simulink model "model_EV_pt1"  (R2022a)
settings: Solver=ode15s  StartTime=0.0  StopTime=tstop  MaxStep=0.001  RelTol=1e-3  EnableMultiTasking=on
undefined symbols (not defined in the file): D, F0, F1, F2, J, Km, La, M, Q, Qo, r_wheel, Ra, Rbatt, slope, SOC_max, SOC_min, Voc, xdot_o
libraries: fl_lib x38, nesl_utility x21, simulink x2, sdl_lib x1
settings Model: Creator=MathWorks  LastModifiedBy=cdjaolek
settings SolverCC: ZeroCrossControl=DisableAll  AlgebraicLoopSolver=TrustRegion
settings DataIOCC: LimitDataPoints=on  SaveFormat=Array  ReturnWorkspaceOutputs=off
settings OptimizationCC: ExpressionDepthLimit=2147483647  InitFltsAndDblsToZero=on  LifeSpan=inf
settings DebuggingCC: AlgebraicLoopMsg=none  SaveWithParameterizedLinksMsg=none  UnderspecifiedInitializationDetection=Classic  MergeDetectMultiDrivingBlocksExec=none  SignalResolutionControl=TryResolveAllWithWarning  SolverPrmCheckMsg=warning  UnconnectedInputMsg=warning  UnconnectedOutputMsg=warning  UnconnectedLineMsg=warning  StateNameClashWarn=warning  SFUnexpectedBacktrackingDiag=warning  SFNoUnconditionalDefaultTransitionDiag=warning  SFExecutionAtInitializationDiag=none  SFMachineParentedDataDiag=warning  ArithmeticOperatorsInVariantConditions=warning
settings HardwareCC: ProdBitPerPointer=32  ProdBitPerSizeT=32  ProdBitPerPtrDiffT=32  ProdLargestAtomicFloat=None  ProdIntDivRoundTo=Undefined  ProdEndianess=Unspecified  ProdWordSize=32  ProdHWDeviceType=32-bit Generic
settings ModelReferenceCC: PropagateSignalLabelsOutOfModel=off
settings SFSimCC: SimUseLocalCustomCode=off  CustomCodeUndefinedFunction=UseInterfaceOnly
settings RTWCC: RTWUseLocalCustomCode=off
settings CodeAppCC: StateflowObjectComments=on
settings GRTTargetCC: TargetFcnLib=ansi_tfl_tmw.mat  TargetLangStandard=C89/C90 (ANSI)  CombineOutputUpdateFcns=off  GRTInterface=on
settings ConfigComp: CovMetricSettings=dw  CovSaveCumulativeToWorkspaceVar=on  CovSaveSingleToWorkspaceVar=on  CovExternalEMLEnable=off
settings SimscapeCC: SimscapeNormalizeSystem=off

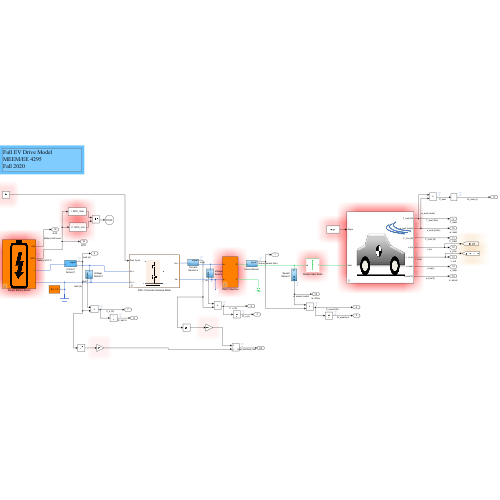
[thumbnail: Simulink's stored preview of the top-level diagram]
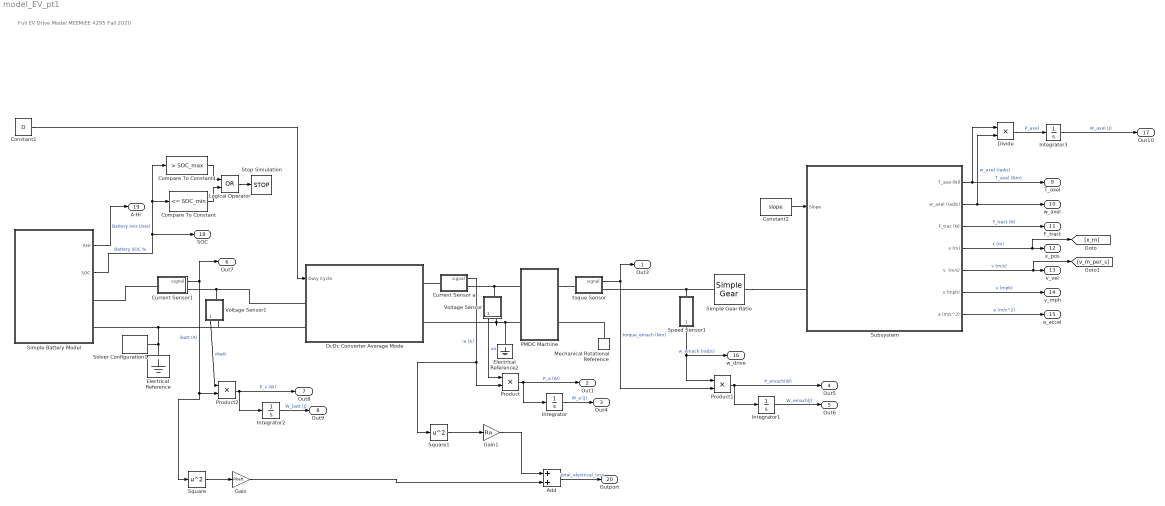
== system model_EV_pt1 ==
  note: Full EV Drive Model
      | MEEM/EE 4295
      | Fall 2020
  Add : Sum
  Compare To Constant : simulink/Logic and Bit Operations/Compare To Constant  relop=<=  const=SOC_min  OutDataTypeStr=boolean
  Compare To Constant1 : simulink/Logic and Bit Operations/Compare To Constant  relop=>  const=SOC_max  OutDataTypeStr=boolean
  Constant1 : Constant  Value=D
  Constant2 : Constant  Value=slope
  Current Sensor a : Subsystem
  Current Sensor1 : Subsystem
  DcDc Converter Average Mode : Subsystem
      mask help: Two Quadrant Dc-Dc convereter - average mode (no switching)
      mask Display: image('$imagefile'); % Use "Edit Image" on toolstrip to change.
  Divide : Product
  Electrical Reference : fl_lib/Electrical/Electrical Elements/Electrical Reference
      settings: SourceProductBaseCode=PW,SS,VE
  Electrical Reference2 : fl_lib/Electrical/Electrical Elements/Electrical Reference
      settings: SourceProductBaseCode=PW,SS,VE
  Gain : Gain  Gain=Rbatt
  Gain1 : Gain  Gain=Ra
  Integrator{,1..3} (4 alike) : Integrator
  Logical Operator : Logic  Operator=OR  AllPortsSameDT=off  OutDataTypeStr=boolean
  Mechanical Rotational Reference : fl_lib/Mechanical/Rotational Elements/Mechanical Rotational Reference
      settings: SourceProductBaseCode=PW,SS,VE
  PMDC Machine : Subsystem  mask{Km=Km, Ra=Ra, La=La, J=J, B=1e-6}
      mask prompts: Km "Motor Constant (Nm/A)"; Ra "Armature Resistance (Ohm)"; La "Armature Inductance (H)"; J "Motor Inertia (kg m^2)"; B "Motor Damping (N*m/(rad/s))"
      mask help: Permanent Magnet DC Motor
  Product : Product
  Product1 : Product
  Product2 : Product
  Simple Battery Model : Subsystem  mask{Voc=Voc, Rbatt=Rbatt, Q=Q, Qo=Qo}
      mask prompts: Voc "Open Circuit Voltage"; Rbatt "Battery  Resistance"; Q "AHr Capacity"; Qo "Initial AHr Used"
      mask help: Simple Battery Model
      mask Display: image('$imagefile'); % Use "Edit Image" on toolstrip to change.
  Simple Gear Ratio : sdl_lib/Gears/Simple Gear  ratio=GR  rotation_direction=3-2*(1)  friction_model=sdl.enum.gear_efficiencies_load.off  T_noload=0.1 N*m  T_nom=5 N*m  efficiency_nom=0.8  efficiency=0.8  temperature_TLU=[280, 300, 320] K  load_TLU=[1, 5, 10] N*m  efficiency_TLU=[.95, .9, .85]  efficiency_TLU2=[.85, .8, .75; .95, .9, .85; .85, .8, .7]  w_thr=0.01 rad/s  pwr_thr=0.001 W  backlash_model=sdl.enum.backlashModel.Off  backlash_distance=1e-3 mm  x0=0 mm  r_base=0.1 m  hardstop_model=simscape.enum.hardstop.smooth  transition=1e-4 mm  backlash_stiffness=1e7 N/m  backlash_damping=1e6 N*s/m  e=0  v_tol=0.001 m/s  mu_visc=[0, 0] N*m/(rad/s)  enable_faults=simscape.enum.onoff.off  efficiency_fault=0.05  external_fault=simscape.enum.onoff.off  temporal_fault=simscape.enum.onoff.off  fault_time=5 s  fault_angles=pi / 12 rad  report_fault=(1)-1  thermal_mass=50 J/K  temperature_specify=off  temperature_priority=High  temperature=300 K  temperature_nominal_specify=off  temperature_nominal_unit=K  temperature_nominal_value=1  x_backlash_specify=off  x_backlash_priority=None  x_backlash=0 mm  x_backlash_nominal_specify=off  x_backlash_nominal_unit=mm  x_backlash_nominal_value=1  f_hardstop_specify=off  f_hardstop_priority=None  f_hardstop=0 N  f_hardstop_nominal_specify=off  f_hardstop_nominal_unit=N  f_hardstop_nominal_value=1  v_backlash_specify=off  v_backlash_priority=None  v_backlash=0 m/s  v_backlash_nominal_specify=off  v_backlash_nominal_unit=m/s  v_backlash_nominal_value=1
  Solver Configuration1 : nesl_utility/Solver Configuration  PhysicalDomain=network_engine_domain  SubClassName=solver  LeftPortType=input  RightPortType=generic  Tones=[]  Harmonics=[]  SimulateNoise=off  Profile=off  UseLocalSampling=off  EnableSwitchedLinearOptims=on  FrequencyDomain=off  UseCCode=off  RelTol=0.001  AbsTol=1e-06  MinStep=1e-09  ToWorkspace=off  RevertToSquareIcSolve=off  NumHomotopyIterations=100  PhasorMode=off  PhasorModeNumHarmonics=1  IndexReductionMethod=DerivativeReplacement  DoDC=off  ResidualTolerance=1e-9  UseLocalSolver=off  LocalSolverChoice=NE_TRAPEZOIDAL_ADVANCER  LocalSolverSampleTime=1e-7  DoFixedCost=off  MaxNonlinIter=3  MaxModeIter=2  ComputeImpulses=off  ImpulseIterations=2  LinearAlgebra=Sparse  LinearAlgebraNumThread=0  EquationFormulation=NE_TIME_EF  DelaysMemoryBudget=1024  AutomaticFiltering=on  FilteringTimeConstant=0.001  PartitionStorageMethod=AS_NEEDED  PartitionMemoryBudget=1024  PartitionMethod=FAST
      settings: SourceProductBaseCode=SS,PW,VE
  Speed Sensor1 : Subsystem
  Square : Math  Operator=square
  Square1 : Math  Operator=square
  Stop Simulation : Stop
  Subsystem : Subsystem  mask{M=M, r_wheel=r_wheel, F0=F0, F1=F1, F2=F2, xdot_o=xdot_o}
      mask prompts: M "Vehicle Mass (kg)"; r_wheel "Wheel Radius (m)"; F0 "Rolling resistance coefficient, a [N]:"; F1 "Rolling and driveline resistance coefficient, b [N*s/m]:"; F2 "Aerodynamic drag coefficient, c [N*s^2/m^2]:"; xdot_o "Initial velocity, xdot_o [m/s]:"
      mask help: Simple vehicle dynamics model.
      mask Display: image('$imagefile'); % Use "Edit Image" on toolstrip to change.
  Voltage Sensor : Subsystem
  Voltage Sensor1 : Subsystem
  toque Sensor : Subsystem
  Out3 : Outport
  Out1 : Outport  Port=2
  Out4 : Outport  Port=3
  Out5 : Outport  Port=4
  Out6 : Outport  Port=5
  Out7 : Outport  Port=6
  Out8 : Outport  Port=7
  Out9 : Outport  Port=8
  T_axel : Outport  Port=9
  w_axel : Outport  Port=10
  F_tract : Outport  Port=11
  x_pos : Outport  Port=12
  v_vel : Outport  Port=13
  v_mph : Outport  Port=14
  a_accel : Outport  Port=15
  w_drive : Outport  Port=16
  Out10 : Outport  Port=17
  SOC : Outport  Port=18
  A-Hr : Outport  Port=19
  Outport : Outport  Port=20
  wires:
  Current Sensor a/1(signal) -> Square1/1, Product/2  "ia (A)"
  toque Sensor/1(signal) -> Out3/1, Product1/2  "torque_emach (Nm)"
  Voltage Sensor/1(signal) -> Product/1  "va"
  Product/1 -> Integrator/1, Out1/1  "P_a (W)"
  Integrator/1 -> Out4/1  "W_a (J)"
  Product1/1 -> Integrator1/1, Out5/1  "P_emach(W)"
  Integrator1/1 -> Out6/1  "W_emach(J)"
  Integrator2/1 -> Out9/1  "W_batt (J)"
  Product2/1 -> Integrator2/1, Out8/1  "P_s (W)"
  Voltage Sensor1/1(signal) -> Product2/1  "vbatt"
  Current Sensor1/1(signal) -> Out7/1, Square/1, Product2/2  "ibatt (A)"
  Constant1/1 -> DcDc Converter Average Mode/1(Duty Cycle)
  Speed Sensor1/1(rad/s) -> Product1/1, w_drive/1  "w_emach (rad/s)"
  Subsystem/2(w_axel (rad/s)) -> w_axel/1, Divide/2  "w_axel (rad/s)"
  Constant2/1 -> Subsystem/1(Slope)
  Subsystem/5(v  (m/s)) -> [v_m_per_s], v_vel/1  "v (m/s)"
  Subsystem/6(v (mph)) -> v_mph/1  "v (mph)"
  Subsystem/1(T_axe (N)l) -> T_axel/1, Divide/1  "T_axel (Nm)"
  Subsystem/3(F_trac (N)) -> F_tract/1  "F_tract (N)"
  Divide/1 -> Integrator3/1  "P_axel"
  Integrator3/1 -> Out10/1  "W_axel (J)"
  Subsystem/7(a (m/s^2)) -> a_accel/1  "a (m/s^2)"
  Subsystem/4(x (m)) -> [x_m], x_pos/1  "x (m)"
  Simple Battery Model/1(AHr) -> A-Hr/1  "Battery AHr Used"
  Logical Operator/1 -> Stop Simulation/1
  Compare To Constant1/1 -> Logical Operator/1
  Simple Battery Model/2(SOC) -> Compare To Constant/1, Compare To Constant1/1, SOC/1  "Battery SOC %"
  Compare To Constant/1 -> Logical Operator/2
  Add/1 -> Outport/1  "total_electrical_loss"
  Square/1 -> Gain/1
  Square1/1 -> Gain1/1
  Gain/1 -> Add/2
  Gain1/1 -> Add/1
  connections:
  Mechanical Rotational Reference/LConn1 -- PMDC Machine/RConn2
  Voltage Sensor/LConn1 -- PMDC Machine/LConn1 -- Current Sensor a/RConn1
  PMDC Machine/RConn1 -- toque Sensor/LConn1
  Solver Configuration1/RConn1 -- Electrical Reference/LConn1 -- Voltage Sensor1/RConn1 -- DcDc Converter Average Mode/LConn2 -- Simple Battery Model/RConn2
  Current Sensor a/LConn1 -- DcDc Converter Average Mode/RConn1
  Current Sensor1/LConn1 -- Simple Battery Model/RConn1
  DcDc Converter Average Mode/LConn1 -- Voltage Sensor1/LConn1 -- Current Sensor1/RConn1
  PMDC Machine/LConn2 -- Electrical Reference2/LConn1 -- Voltage Sensor/RConn1 -- DcDc Converter Average Mode/RConn2
  Speed Sensor1/LConn1 -- Simple Gear Ratio/LConn1 -- toque Sensor/RConn1
  Simple Gear Ratio/RConn1 -- Subsystem/LConn1

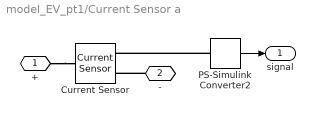
== system model_EV_pt1/Current Sensor a ==
  Current Sensor : fl_lib/Electrical/Electrical Sensors/Current Sensor
      settings: SourceProductBaseCode=PW,SS,VE
  PS-Simulink Converter2 : nesl_utility/PS-Simulink Converter  PhysicalDomain=network_engine_domain  SubClassName=ps_output  LeftPortType=input  RightPortType=output  PseudoPeriodic=off  Frequencies=[]  VectorFormat=1-D array  Unit=1  AffineConversion=off
      settings: SourceProductBaseCode=SS,PW,VE
  + : PMIOPort  Side=Left
  - : PMIOPort  Port=2  Side=Right
  signal : Outport
  wires:
  PS-Simulink Converter2/1 -> signal/1
  connections:
  PS-Simulink Converter2/LConn1 -- Current Sensor/RConn1
  +/RConn1 -- Current Sensor/LConn1
  -/RConn1 -- Current Sensor/RConn2

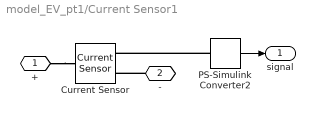
== system model_EV_pt1/Current Sensor1 ==
  Current Sensor : fl_lib/Electrical/Electrical Sensors/Current Sensor
      settings: SourceProductBaseCode=PW,SS,VE
  PS-Simulink Converter2 : nesl_utility/PS-Simulink Converter  PhysicalDomain=network_engine_domain  SubClassName=ps_output  LeftPortType=input  RightPortType=output  PseudoPeriodic=off  Frequencies=[]  VectorFormat=1-D array  Unit=1  AffineConversion=off
      settings: SourceProductBaseCode=SS,PW,VE
  + : PMIOPort  Side=Left
  - : PMIOPort  Port=2  Side=Right
  signal : Outport
  wires:
  PS-Simulink Converter2/1 -> signal/1
  connections:
  PS-Simulink Converter2/LConn1 -- Current Sensor/RConn1
  +/RConn1 -- Current Sensor/LConn1
  -/RConn1 -- Current Sensor/RConn2

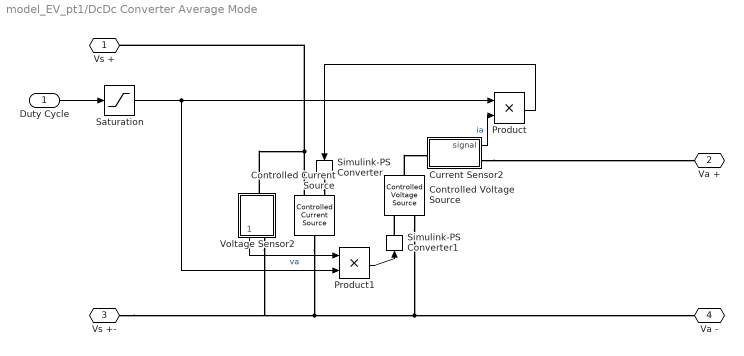
== system model_EV_pt1/DcDc Converter Average Mode ==
  Duty Cycle : Inport
  Controlled Current Source : fl_lib/Electrical/Electrical Sources/Controlled Current Source
      settings: SourceProductBaseCode=PW,SS,VE
  Controlled Voltage Source : fl_lib/Electrical/Electrical Sources/Controlled Voltage Source
      settings: SourceProductBaseCode=PW,SS,VE
  Current Sensor2 : Subsystem
  Product : Product
  Product1 : Product
  Saturation : Saturate  UpperLimit=1  LowerLimit=0
  Simulink-PS Converter : nesl_utility/Simulink-PS Converter  PhysicalDomain=network_engine_domain  SubClassName=ps_input  LeftPortType=input  RightPortType=output  PseudoPeriodic=off  Frequencies=[]  NoiseDistribution=none  NoiseParameters=[]  Unit=1  AffineConversion=off  FilteringAndDerivatives=provide  SimscapeFilterOrder=1  InputFilterTimeConstant=0.001  UdotUserProvided=0
      settings: SourceProductBaseCode=SS,PW,VE
  Simulink-PS Converter1 : nesl_utility/Simulink-PS Converter  PhysicalDomain=network_engine_domain  SubClassName=ps_input  LeftPortType=input  RightPortType=output  PseudoPeriodic=off  Frequencies=[]  NoiseDistribution=none  NoiseParameters=[]  Unit=1  AffineConversion=off  FilteringAndDerivatives=provide  SimscapeFilterOrder=1  InputFilterTimeConstant=0.001  UdotUserProvided=0
      settings: SourceProductBaseCode=SS,PW,VE
  Voltage Sensor2 : Subsystem
  Vs + : PMIOPort  Side=Left
  Va + : PMIOPort  Port=2  Side=Right
  Vs +- : PMIOPort  Port=3  Side=Left
  Va - : PMIOPort  Port=4  Side=Right
  wires:
  Product1/1 -> Simulink-PS Converter1/1
  Duty Cycle/1 -> Saturation/1
  Voltage Sensor2/1(signal) -> Product1/1  "va"
  Product/1 -> Simulink-PS Converter/1
  Current Sensor2/1(signal) -> Product/2  "ia"
  Saturation/1 -> Product1/2, Product/1
  connections:
  Controlled Current Source/RConn2 -- Vs +/RConn1 -- Voltage Sensor2/LConn1
  Simulink-PS Converter/RConn1 -- Controlled Current Source/RConn1
  Simulink-PS Converter1/RConn1 -- Controlled Voltage Source/RConn1
  Controlled Voltage Source/LConn1 -- Current Sensor2/LConn1
  Current Sensor2/RConn1 -- Va +/RConn1
  Controlled Voltage Source/RConn2 -- Voltage Sensor2/RConn1 -- Vs +-/RConn1 -- Controlled Current Source/LConn1 -- Va -/RConn1

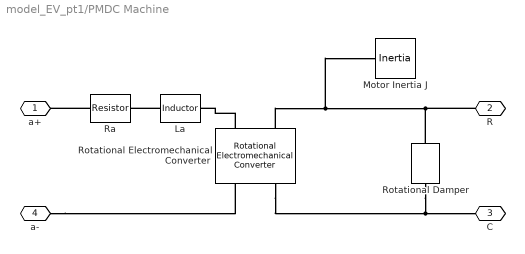
== system model_EV_pt1/PMDC Machine ==
  La : fl_lib/Electrical/Electrical Elements/Inductor  l=La H  r=0 Ohm  g=1e-09 1/Ohm  i_specify=off  i_priority=None  i=0 A  i_nominal_specify=off  i_nominal_unit=A  i_nominal_value=1  v_specify=off  v_priority=None  v=0 V  v_nominal_specify=off  v_nominal_unit=V  v_nominal_value=1  i_L_specify=on  i_L_priority=High  i_L=0 A  i_L_nominal_specify=off  i_L_nominal_unit=A  i_L_nominal_value=1
      settings: SourceProductBaseCode=PW,SS,VE
  Motor Inertia J : fl_lib/Mechanical/Rotational Elements/Inertia  inertia=J kg*m^2  num_ports=foundation.enum.numPorts2.one  w_specify=on  w_priority=High  w=0 rad/s  w_nominal_specify=off  w_nominal_unit=rad/s  w_nominal_value=1  t_specify=off  t_priority=None  t=0 N*m  t_nominal_specify=off  t_nominal_unit=N*m  t_nominal_value=1
      settings: SourceProductBaseCode=PW,SS,VE
  Ra : fl_lib/Electrical/Electrical Elements/Resistor  Tag=Factory Generic  R=Ra Ohm  i_specify=off  i_priority=None  i=0 A  i_nominal_specify=off  i_nominal_unit=A  i_nominal_value=1  v_specify=off  v_priority=None  v=0 V  v_nominal_specify=off  v_nominal_unit=V  v_nominal_value=1
      settings: SourceProductBaseCode=PW,SS,VE
  Rotational Damper : fl_lib/Mechanical/Rotational Elements/Rotational Damper  D=B N*m/(rad/s)  w_specify=off  w_priority=None  w=0 rad/s  w_nominal_specify=off  w_nominal_unit=rad/s  w_nominal_value=1  t_specify=off  t_priority=None  t=0 N*m  t_nominal_specify=off  t_nominal_unit=N*m  t_nominal_value=1
      settings: SourceProductBaseCode=PW,SS,VE
  Rotational Electromechanical Converter : fl_lib/Electrical/Electrical Elements/Rotational Electromechanical Converter  K=Km V/(rad/s)  i_specify=off  i_priority=None  i=0 A  i_nominal_specify=off  i_nominal_unit=A  i_nominal_value=1  v_specify=off  v_priority=None  v=0 V  v_nominal_specify=off  v_nominal_unit=V  v_nominal_value=1  t_specify=off  t_priority=None  t=0 N*m  t_nominal_specify=off  t_nominal_unit=N*m  t_nominal_value=1  w_specify=off  w_priority=None  w=0 rad/s  w_nominal_specify=off  w_nominal_unit=rad/s  w_nominal_value=1
      settings: SourceProductBaseCode=PW,SS,VE
  a+ : PMIOPort  Side=Left
  R : PMIOPort  Port=2  Side=Right
  C : PMIOPort  Port=3  Side=Right
  a- : PMIOPort  Port=4  Side=Left
  connections:
  Rotational Electromechanical Converter/LConn1 -- La/RConn1
  a-/RConn1 -- Rotational Electromechanical Converter/RConn1
  Ra/LConn1 -- a+/RConn1
  La/LConn1 -- Ra/RConn1
  Rotational Electromechanical Converter/LConn2 -- Motor Inertia J/LConn1 -- R/RConn1 -- Rotational Damper/LConn1
  Rotational Electromechanical Converter/RConn2 -- C/RConn1 -- Rotational Damper/RConn1

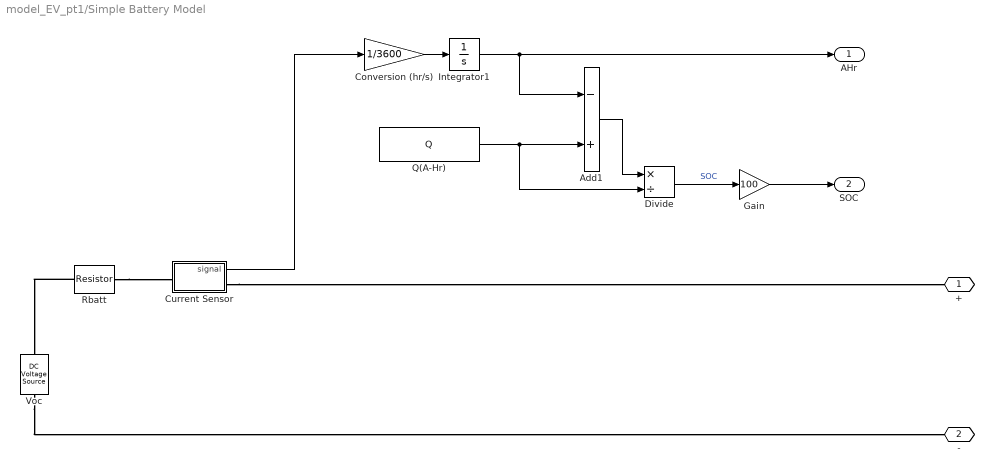
== system model_EV_pt1/Simple Battery Model ==
  Add1 : Sum  Inputs=-+
  Conversion (hr/s) : Gain  Gain=1/3600
  Current Sensor : Subsystem
  Divide : Product  Inputs=*/
  Gain : Gain  Gain=100
  Integrator1 : Integrator  InitialCondition=Qo  UpperSaturationLimit=Q*1.5  LowerSaturationLimit=0
  Q(A-Hr) : Constant  Value=Q
  Rbatt : fl_lib/Electrical/Electrical Elements/Resistor  R=Rbatt Ohm  i_specify=off  i_priority=None  i=0 A  i_nominal_specify=off  i_nominal_unit=A  i_nominal_value=1  v_specify=off  v_priority=None  v=0 V  v_nominal_specify=off  v_nominal_unit=V  v_nominal_value=1
      settings: SourceProductBaseCode=PW,SS,VE
  Voc : fl_lib/Electrical/Electrical Sources/DC Voltage Source  v0=Voc V
      settings: SourceProductBaseCode=PW,SS,VE
  + : PMIOPort  Side=Right
  - : PMIOPort  Port=2  Side=Right
  AHr : Outport
  SOC : Outport  Port=2
  wires:
  Integrator1/1 -> AHr/1, Add1/1
  Conversion (hr/s)/1 -> Integrator1/1
  Add1/1 -> Divide/1
  Divide/1 -> Gain/1  "SOC"
  Q(A-Hr)/1 -> Add1/2, Divide/2
  Gain/1 -> SOC/1
  Current Sensor/1(signal) -> Conversion (hr/s)/1
  connections:
  Rbatt/RConn1 -- Current Sensor/LConn1
  Current Sensor/RConn1 -- +/RConn1
  Rbatt/LConn1 -- Voc/LConn1
  Voc/RConn1 -- -/RConn1

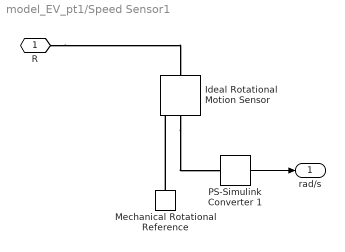
== system model_EV_pt1/Speed Sensor1 ==
  Ideal Rotational Motion Sensor : fl_lib/Mechanical/Mechanical Sensors/Ideal Rotational Motion Sensor  wrap_angle=simscape.enum.onoff.off  offset=0 rad
      settings: SourceProductBaseCode=PW,SS,VE
  Mechanical Rotational Reference : fl_lib/Mechanical/Rotational Elements/Mechanical Rotational Reference
      settings: SourceProductBaseCode=PW,SS,VE
  PS-Simulink Converter 1 : nesl_utility/PS-Simulink Converter  PhysicalDomain=network_engine_domain  SubClassName=ps_output  LeftPortType=input  RightPortType=output  PseudoPeriodic=off  Frequencies=[]  VectorFormat=1-D array  Unit=rad/s  AffineConversion=off
      settings: SourceProductBaseCode=SS,PW,VE
  R : PMIOPort  Side=Left
  rad/s : Outport
  wires:
  PS-Simulink Converter 1/1 -> rad/s/1
  connections:
  Ideal Rotational Motion Sensor/RConn2 -- PS-Simulink Converter 1/LConn1
  R/RConn1 -- Ideal Rotational Motion Sensor/LConn1
  Mechanical Rotational Reference/LConn1 -- Ideal Rotational Motion Sensor/RConn1

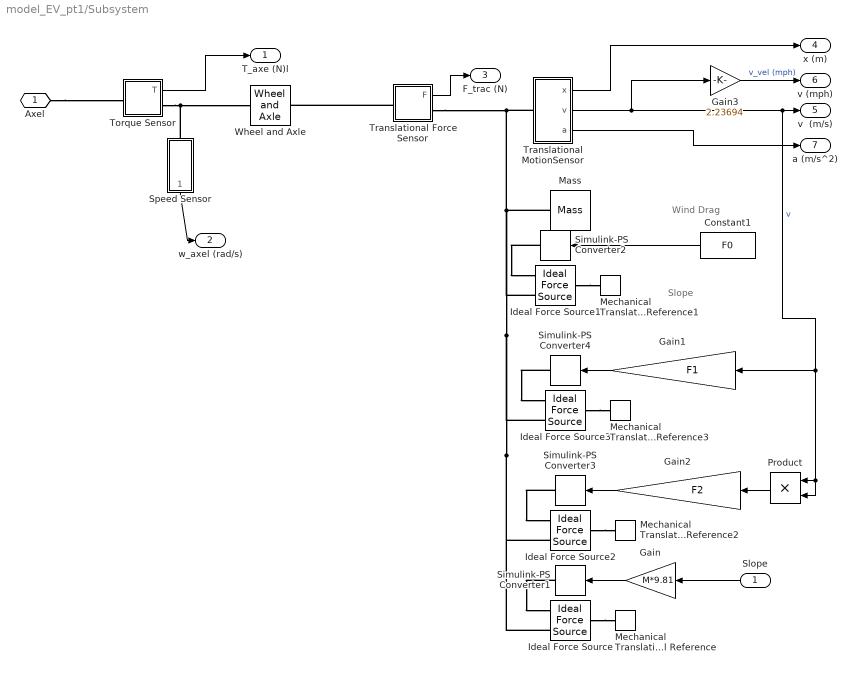
== system model_EV_pt1/Subsystem ==
  note: Wind Drag
  note: Slope
  Slope : Inport
  Constant1 : Constant  Value=F0
  Gain : Gain  Gain=M*9.81
  Gain1 : Gain  Gain=F1
  Gain2 : Gain  Gain=F2
  Gain3 : Gain  Gain=2.23694
  Ideal Force Source{,1..3} (4 alike) : fl_lib/Mechanical/Mechanical Sources/Ideal Force Source
      settings: SourceProductBaseCode=PW,SS,VE
  Mass : fl_lib/Mechanical/Translational Elements/Mass  mass=M kg  num_ports=foundation.enum.numPorts2.one  v_specify=on  v_priority=High  v=xdot_o m/s  v_nominal_specify=off  v_nominal_unit=m/s  v_nominal_value=1  f_specify=off  f_priority=None  f=0 N  f_nominal_specify=off  f_nominal_unit=N  f_nominal_value=1
      settings: SourceProductBaseCode=PW,SS,VE
  Mechanical Translational Reference{,1..3} (4 alike) : fl_lib/Mechanical/Translational Elements/Mechanical Translational Reference
      settings: SourceProductBaseCode=PW,SS,VE
  Product : Product  RndMeth=Zero
  Simulink-PS Converter{1..4} (4 alike) : nesl_utility/Simulink-PS Converter  PhysicalDomain=network_engine_domain  SubClassName=ps_input  LeftPortType=input  RightPortType=output  PseudoPeriodic=off  Frequencies=[]  NoiseDistribution=none  NoiseParameters=[]  Unit=1  AffineConversion=off  FilteringAndDerivatives=zero  SimscapeFilterOrder=1  InputFilterTimeConstant=.001  UdotUserProvided=[]
      settings: SourceProductBaseCode=SS,PW,VE
  Speed Sensor : Subsystem
  Torque Sensor : Subsystem
  Translational Force Sensor : Subsystem
  Translational MotionSensor : Subsystem
  Wheel and Axle : fl_lib/Mechanical/Mechanisms/Wheel and Axle  Tag=Factory Generic  R=r_wheel m  or=1  t_specify=off  t_priority=None  t=0 N*m  t_nominal_specify=off  t_nominal_unit=N*m  t_nominal_value=1  f_specify=off  f_priority=None  f=0 N  f_nominal_specify=off  f_nominal_unit=N  f_nominal_value=1
      settings: SourceProductBaseCode=PW,SS,VE
  Axel : PMIOPort  Side=Left
  T_axe (N)l : Outport
  w_axel (rad/s) : Outport  Port=2
  F_trac (N) : Outport  Port=3
  x (m) : Outport  Port=4
  v  (m/s) : Outport  Port=5
  v (mph) : Outport  Port=6
  a (m/s^2) : Outport  Port=7
  wires:
  Product/1 -> Gain2/1
  Translational MotionSensor/2(v) -> Gain1/1, Product/2, Product/1, v  (m/s)/1, Gain3/1  "v"
  Speed Sensor/1(rad/s) -> w_axel (rad/s)/1
  Gain/1 -> Simulink-PS Converter1/1
  Gain2/1 -> Simulink-PS Converter3/1
  Torque Sensor/1(T) -> T_axe (N)l/1
  Translational MotionSensor/1(x) -> x (m)/1
  Translational MotionSensor/3(a) -> a (m/s^2)/1
  Translational Force Sensor/1(F) -> F_trac (N)/1
  Slope/1 -> Gain/1
  Gain3/1 -> v (mph)/1  "v_vel (mph)"
  Constant1/1 -> Simulink-PS Converter2/1
  Gain1/1 -> Simulink-PS Converter4/1
  connections:
  Ideal Force Source1/LConn1 -- Mechanical Translational Reference1/LConn1
  Mass/LConn1 -- Ideal Force Source3/RConn2 -- Ideal Force Source/RConn2 -- Ideal Force Source2/RConn2 -- Ideal Force Source1/RConn2 -- Translational MotionSensor/LConn1 -- Translational Force Sensor/RConn1
  Ideal Force Source2/LConn1 -- Mechanical Translational Reference2/LConn1
  Torque Sensor/RConn1 -- Wheel and Axle/LConn1 -- Speed Sensor/LConn1
  Simulink-PS Converter1/RConn1 -- Ideal Force Source/RConn1
  Simulink-PS Converter2/RConn1 -- Ideal Force Source1/RConn1
  Ideal Force Source/LConn1 -- Mechanical Translational Reference/LConn1
  Translational Force Sensor/LConn1 -- Wheel and Axle/RConn1
  Simulink-PS Converter3/RConn1 -- Ideal Force Source2/RConn1
  Axel/RConn1 -- Torque Sensor/LConn1
  Simulink-PS Converter4/RConn1 -- Ideal Force Source3/RConn1
  Ideal Force Source3/LConn1 -- Mechanical Translational Reference3/LConn1

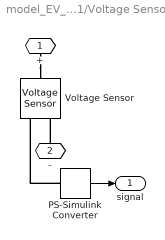
== system model_EV_pt1/Voltage Sensor ==
  PS-Simulink Converter : nesl_utility/PS-Simulink Converter  PhysicalDomain=network_engine_domain  SubClassName=ps_output  LeftPortType=input  RightPortType=output  PseudoPeriodic=off  Frequencies=[]  VectorFormat=1-D array  Unit=1  AffineConversion=off
      settings: SourceProductBaseCode=SS,PW,VE
  Voltage Sensor : fl_lib/Electrical/Electrical Sensors/Voltage Sensor
      settings: SourceProductBaseCode=PW,SS,VE
  + : PMIOPort  Side=Left
  - : PMIOPort  Port=2  Side=Right
  signal : Outport
  wires:
  PS-Simulink Converter/1 -> signal/1
  connections:
  PS-Simulink Converter/LConn1 -- Voltage Sensor/RConn1
  +/RConn1 -- Voltage Sensor/LConn1
  -/RConn1 -- Voltage Sensor/RConn2

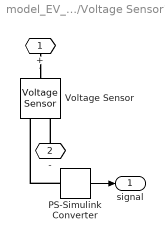
== system model_EV_pt1/Voltage Sensor1 ==
  PS-Simulink Converter : nesl_utility/PS-Simulink Converter  PhysicalDomain=network_engine_domain  SubClassName=ps_output  LeftPortType=input  RightPortType=output  PseudoPeriodic=off  Frequencies=[]  VectorFormat=1-D array  Unit=1  AffineConversion=off
      settings: SourceProductBaseCode=SS,PW,VE
  Voltage Sensor : fl_lib/Electrical/Electrical Sensors/Voltage Sensor
      settings: SourceProductBaseCode=PW,SS,VE
  + : PMIOPort  Side=Left
  - : PMIOPort  Port=2  Side=Right
  signal : Outport
  wires:
  PS-Simulink Converter/1 -> signal/1
  connections:
  PS-Simulink Converter/LConn1 -- Voltage Sensor/RConn1
  +/RConn1 -- Voltage Sensor/LConn1
  -/RConn1 -- Voltage Sensor/RConn2

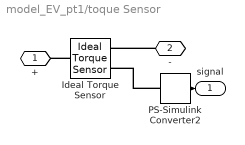
== system model_EV_pt1/toque Sensor ==
  Ideal Torque Sensor : fl_lib/Mechanical/Mechanical Sensors/Ideal Torque Sensor
      settings: SourceProductBaseCode=PW,SS,VE
  PS-Simulink Converter2 : nesl_utility/PS-Simulink Converter  PhysicalDomain=network_engine_domain  SubClassName=ps_output  LeftPortType=input  RightPortType=output  PseudoPeriodic=off  Frequencies=[]  VectorFormat=1-D array  Unit=1  AffineConversion=off
      settings: SourceProductBaseCode=SS,PW,VE
  + : PMIOPort  Side=Left
  - : PMIOPort  Port=2  Side=Right
  signal : Outport
  wires:
  PS-Simulink Converter2/1 -> signal/1
  connections:
  Ideal Torque Sensor/LConn1 -- +/RConn1
  -/RConn1 -- Ideal Torque Sensor/RConn1
  PS-Simulink Converter2/LConn1 -- Ideal Torque Sensor/RConn2

== system model_EV_pt1/DcDc Converter Average Mode/Current Sensor2 ==
  Current Sensor : fl_lib/Electrical/Electrical Sensors/Current Sensor
      settings: SourceProductBaseCode=PW,SS,VE
  PS-Simulink Converter2 : nesl_utility/PS-Simulink Converter  PhysicalDomain=network_engine_domain  SubClassName=ps_output  LeftPortType=input  RightPortType=output  PseudoPeriodic=off  Frequencies=[]  VectorFormat=1-D array  Unit=1  AffineConversion=off
      settings: SourceProductBaseCode=SS,PW,VE
  + : PMIOPort  Side=Left
  - : PMIOPort  Port=2  Side=Right
  signal : Outport
  wires:
  PS-Simulink Converter2/1 -> signal/1
  connections:
  PS-Simulink Converter2/LConn1 -- Current Sensor/RConn1
  +/RConn1 -- Current Sensor/LConn1
  -/RConn1 -- Current Sensor/RConn2

== system model_EV_pt1/DcDc Converter Average Mode/Voltage Sensor2 ==
  PS-Simulink Converter : nesl_utility/PS-Simulink Converter  PhysicalDomain=network_engine_domain  SubClassName=ps_output  LeftPortType=input  RightPortType=output  PseudoPeriodic=off  Frequencies=[]  VectorFormat=1-D array  Unit=1  AffineConversion=off
      settings: SourceProductBaseCode=SS,PW,VE
  Voltage Sensor : fl_lib/Electrical/Electrical Sensors/Voltage Sensor
      settings: SourceProductBaseCode=PW,SS,VE
  + : PMIOPort  Side=Left
  - : PMIOPort  Port=2  Side=Right
  signal : Outport
  wires:
  PS-Simulink Converter/1 -> signal/1
  connections:
  PS-Simulink Converter/LConn1 -- Voltage Sensor/RConn1
  +/RConn1 -- Voltage Sensor/LConn1
  -/RConn1 -- Voltage Sensor/RConn2

== system model_EV_pt1/Simple Battery Model/Current Sensor ==
  Current Sensor : fl_lib/Electrical/Electrical Sensors/Current Sensor
      settings: SourceProductBaseCode=PW,SS,VE
  PS-Simulink Converter2 : nesl_utility/PS-Simulink Converter  PhysicalDomain=network_engine_domain  SubClassName=ps_output  LeftPortType=input  RightPortType=output  PseudoPeriodic=off  Frequencies=[]  VectorFormat=1-D array  Unit=1  AffineConversion=off
      settings: SourceProductBaseCode=SS,PW,VE
  + : PMIOPort  Side=Left
  - : PMIOPort  Port=2  Side=Right
  signal : Outport
  wires:
  PS-Simulink Converter2/1 -> signal/1
  connections:
  PS-Simulink Converter2/LConn1 -- Current Sensor/RConn1
  +/RConn1 -- Current Sensor/LConn1
  -/RConn1 -- Current Sensor/RConn2

== system model_EV_pt1/Subsystem/Speed Sensor ==
  Ideal Rotational Motion Sensor : fl_lib/Mechanical/Mechanical Sensors/Ideal Rotational Motion Sensor  wrap_angle=simscape.enum.onoff.off  offset=0 rad
      settings: SourceProductBaseCode=PW,SS,VE
  Mechanical Rotational Reference : fl_lib/Mechanical/Rotational Elements/Mechanical Rotational Reference
      settings: SourceProductBaseCode=PW,SS,VE
  PS-Simulink Converter 1 : nesl_utility/PS-Simulink Converter  PhysicalDomain=network_engine_domain  SubClassName=ps_output  LeftPortType=input  RightPortType=output  PseudoPeriodic=off  Frequencies=[]  VectorFormat=1-D array  Unit=rad/s  AffineConversion=off
      settings: SourceProductBaseCode=SS,PW,VE
  R : PMIOPort  Side=Left
  rad/s : Outport
  wires:
  PS-Simulink Converter 1/1 -> rad/s/1
  connections:
  Ideal Rotational Motion Sensor/RConn2 -- PS-Simulink Converter 1/LConn1
  R/RConn1 -- Ideal Rotational Motion Sensor/LConn1
  Mechanical Rotational Reference/LConn1 -- Ideal Rotational Motion Sensor/RConn1

== system model_EV_pt1/Subsystem/Torque Sensor ==
  Ideal Torque Sensor : fl_lib/Mechanical/Mechanical Sensors/Ideal Torque Sensor
      settings: SourceProductBaseCode=PW,SS,VE
  PS-Simulink Converter1 : nesl_utility/PS-Simulink Converter  PhysicalDomain=network_engine_domain  SubClassName=ps_output  LeftPortType=input  RightPortType=output  PseudoPeriodic=off  Frequencies=[]  VectorFormat=1-D array  Unit=1  AffineConversion=off
      settings: SourceProductBaseCode=SS,PW,VE
  R : PMIOPort  Side=Left
  C : PMIOPort  Port=2  Side=Right
  T : Outport
  wires:
  PS-Simulink Converter1/1 -> T/1
  connections:
  Ideal Torque Sensor/LConn1 -- R/RConn1
  Ideal Torque Sensor/RConn1 -- C/RConn1
  Ideal Torque Sensor/RConn2 -- PS-Simulink Converter1/LConn1

== system model_EV_pt1/Subsystem/Translational Force Sensor ==
  Ideal Force Sensor : fl_lib/Mechanical/Mechanical Sensors/Ideal Force Sensor
      settings: SourceProductBaseCode=PW,SS,VE
  PS-Simulink Converter1 : nesl_utility/PS-Simulink Converter  PhysicalDomain=network_engine_domain  SubClassName=ps_output  LeftPortType=input  RightPortType=output  PseudoPeriodic=off  Frequencies=[]  VectorFormat=1-D array  Unit=1  AffineConversion=off
      settings: SourceProductBaseCode=SS,PW,VE
  R : PMIOPort  Side=Left
  C : PMIOPort  Port=2  Side=Right
  F : Outport
  wires:
  PS-Simulink Converter1/1 -> F/1
  connections:
  Ideal Force Sensor/LConn1 -- R/RConn1
  Ideal Force Sensor/RConn1 -- C/RConn1
  PS-Simulink Converter1/LConn1 -- Ideal Force Sensor/RConn2

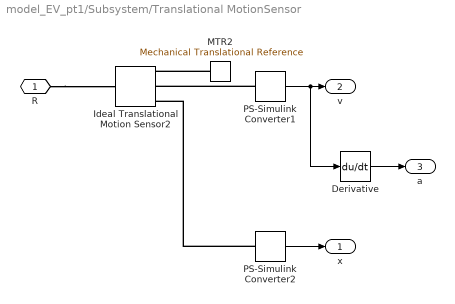
== system model_EV_pt1/Subsystem/Translational MotionSensor ==
  Derivative : Derivative
  Ideal Translational Motion Sensor2 : fl_lib/Mechanical/Mechanical Sensors/Ideal Translational Motion Sensor  Tag=Factory Generic  offset=0 m
      settings: SourceProductBaseCode=PW,SS,VE
  MTR2 : fl_lib/Mechanical/Translational Elements/Mechanical Translational Reference  Tag=Factory Generic
      settings: SourceProductBaseCode=PW,SS,VE
  PS-Simulink Converter1 : nesl_utility/PS-Simulink Converter  PhysicalDomain=network_engine_domain  SubClassName=ps_output  LeftPortType=input  RightPortType=output  PseudoPeriodic=off  Frequencies=[]  VectorFormat=1-D array  Unit=1  AffineConversion=off
      settings: SourceProductBaseCode=SS,PW,VE
  PS-Simulink Converter2 : nesl_utility/PS-Simulink Converter  PhysicalDomain=network_engine_domain  SubClassName=ps_output  LeftPortType=input  RightPortType=output  PseudoPeriodic=off  Frequencies=[]  VectorFormat=1-D array  Unit=1  AffineConversion=off
      settings: SourceProductBaseCode=SS,PW,VE
  R : PMIOPort  Side=Left
  x : Outport
  v : Outport  Port=2
  a : Outport  Port=3
  wires:
  PS-Simulink Converter2/1 -> x/1
  PS-Simulink Converter1/1 -> Derivative/1, v/1
  Derivative/1 -> a/1
  connections:
  MTR2/LConn1 -- Ideal Translational Motion Sensor2/RConn1
  PS-Simulink Converter2/LConn1 -- Ideal Translational Motion Sensor2/RConn3
  R/RConn1 -- Ideal Translational Motion Sensor2/LConn1
  PS-Simulink Converter1/LConn1 -- Ideal Translational Motion Sensor2/RConn2
